simulink model "tf_hex_pos"  (R2020a)
settings: Solver=FixedStepAuto  StartTime=0.0  StopTime=10.0  FixedStep=step_size  RelTol=1e-3
values from neighbouring files (symbols this model uses):
  A = diag([Ax Ax Ax])    [tf_model_sim.m]
  g = 9.81    [tf_model_sim.m]
  m = 1.89    [tf_model_sim.m]
  pitch_tf = tf([omega_n^2], [1 2*zeta*omega_n omega_n^2])*tf([pl],[1 pl],'InputDelay',0.09)    [tf_model_sim.m]
  Ts = 0.01    [tf_model_sim.m]
undefined symbols (not defined in the file or in its folder): kd, ki, kp
settings Model: Creator=pala  LastModifiedBy=pala
settings DataIOCC: SaveFormat=StructureWithTime  ReturnWorkspaceOutputs=off

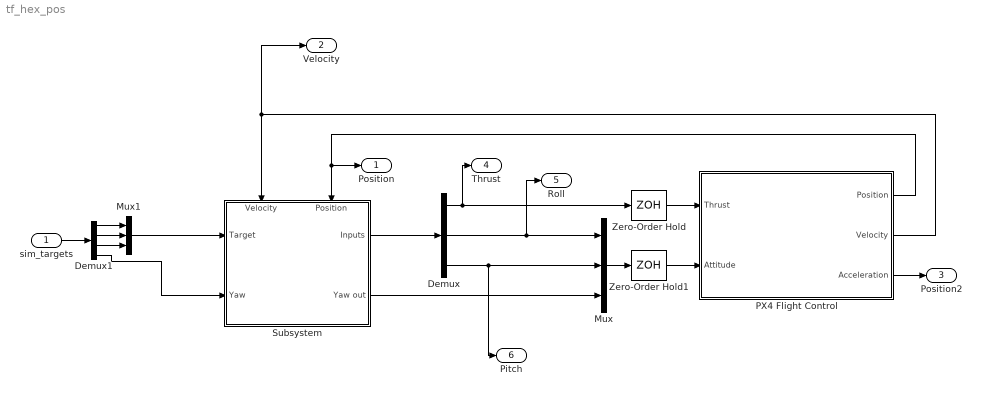
== system tf_hex_pos ==
  sim_targets : Inport
  Demux : Demux  Outputs=3
  Demux1 : Demux
  Mux : Mux  Inputs=3
  Mux1 : Mux  Inputs=3
  PX4 Flight Control : Subsystem
  Subsystem : Subsystem
      settings: PortSchema="{\"entries\":[{\"content\":{\"sides\":[{\"content\":{\"connectorIds\":[\"In1\",\"In2\"]},\"type\":\"ConnectorPlacement.EquallySpacedRectSide\",\"uuid\":\"741a1eff-fa24-40e3-8584-656dcfb9063f\"},{\"content\":{\"connectorIds\":[\"Out1\",\"Out2\"],\"side\":\"RIGHT\"},\"type\":\"ConnectorPlacement.EquallySpacedRectSide\",\"uuid\":\"ed08c2cd-e579-42d0-ad38-ef4d944c32e6\"},{\"content\":{\"connectorIds\":[\"In3\",\"In4\"],\"side\":\"TOP\"},\"type\":\"ConnectorPlacement.EquallySpacedRectSide\",\"uuid\":\"8a6d1a88-6848-4266-a6d4-735010b8417e\"}]},\"type\":\"ConnectorPlacement.EquallySpacedConnector\",\"uuid\":\"0638f19b-f024-4dd2-b120-329a1c216fc8\"}],\"packageUris\":[\"http://schema.mathworks.com/mf0/Connector/19700101\"],\"version\":\"1.0\"}"
  Zero-Order Hold : ZeroOrderHold  SampleTime=Ts
  Zero-Order Hold1 : ZeroOrderHold  SampleTime=Ts
  Position : Outport
  Velocity : Outport  Port=2
  Position2 : Outport  Port=3
  Thrust : Outport  Port=4
  Roll : Outport  Port=5
  Pitch : Outport  Port=6
  wires:
  Demux/3 -> Pitch/1, Mux/2
  Demux/2 -> Roll/1, Mux/1
  Demux/1 -> Zero-Order Hold/1, Thrust/1
  Mux/1 -> Zero-Order Hold1/1
  PX4 Flight Control/1(Position) -> Position/1, Subsystem/4(Position)
  Mux1/1 -> Subsystem/1(Target)
  PX4 Flight Control/2(Velocity) -> Velocity/1, Subsystem/3(Velocity)
  Demux1/4 -> Subsystem/2(Yaw)
  Subsystem/1(Inputs) -> Demux/1
  Subsystem/2(Yaw out) -> Mux/3
  sim_targets/1 -> Demux1/1
  Demux1/1 -> Mux1/1
  Demux1/2 -> Mux1/2
  Demux1/3 -> Mux1/3
  PX4 Flight Control/3(Acceleration) -> Position2/1
  Zero-Order Hold1/1 -> PX4 Flight Control/2(Attitude)
  Zero-Order Hold/1 -> PX4 Flight Control/1(Thrust)

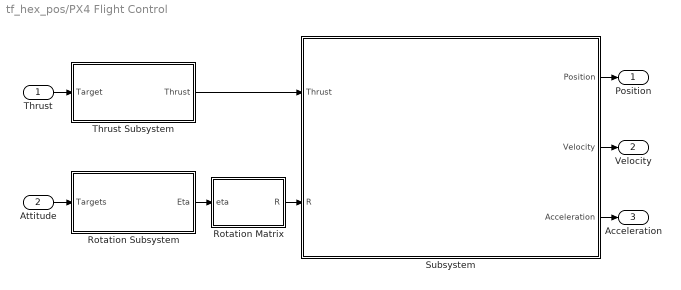
== system tf_hex_pos/PX4 Flight Control ==
  Thrust : Inport
  Attitude : Inport  Port=2
  Rotation Matrix : MATLAB Function  TreatAsAtomicUnit=on
  Rotation Subsystem : Subsystem
  Subsystem : Subsystem
  Thrust Subsystem : Subsystem
  Position : Outport
  Velocity : Outport  Port=2
  Acceleration : Outport  Port=3
  wires:
  Rotation Subsystem/1(Eta) -> Rotation Matrix/1(eta)
  Rotation Matrix/1(R) -> Subsystem/2(R)
  Subsystem/3(Acceleration) -> Acceleration/1
  Thrust/1 -> Thrust Subsystem/1(Target)
  Thrust Subsystem/1(Thrust) -> Subsystem/1(Thrust)
  Subsystem/1(Position) -> Position/1
  Subsystem/2(Velocity) -> Velocity/1
  Attitude/1 -> Rotation Subsystem/1(Targets)

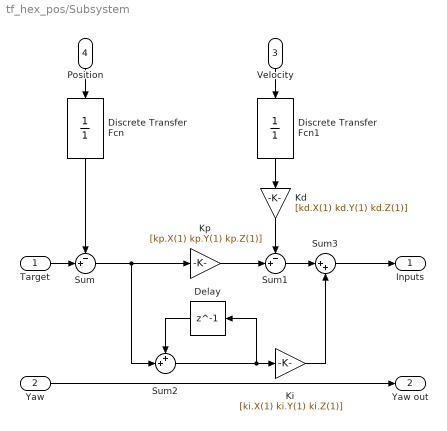
== system tf_hex_pos/Subsystem ==
  Target : Inport
  Yaw : Inport  Port=2
  Velocity : Inport  Port=3
  Position : Inport  Port=4
  Delay : Delay  DelayLength=1  SampleTime=Ts
  Discrete Transfer Fcn : DiscreteTransferFcn  Denominator=[1]  SampleTime=Ts
  Discrete Transfer Fcn1 : DiscreteTransferFcn  Denominator=[1]  SampleTime=Ts
  Kd : Gain  Gain=[kd.X(1) kd.Y(1) kd.Z(1)]
  Ki : Gain  Gain=[ki.X(1) ki.Y(1) ki.Z(1)]
  Kp : Gain  Gain=[kp.X(1) kp.Y(1) kp.Z(1)]
  Sum : Sum  Inputs=-+|
  Sum1 : Sum  Inputs=-+|
  Sum2 : Sum  Inputs=++|
  Sum3 : Sum  Inputs=|++
  Inputs : Outport
  Yaw out : Outport  Port=2
  wires:
  Target/1 -> Sum/2
  Kd/1 -> Sum1/1
  Ki/1 -> Sum3/2
  Sum/1 -> Kp/1, Sum2/2
  Position/1 -> Discrete Transfer Fcn/1
  Velocity/1 -> Discrete Transfer Fcn1/1
  Yaw/1 -> Yaw out/1
  Kp/1 -> Sum1/2
  Sum2/1 -> Ki/1, Delay/1
  Discrete Transfer Fcn1/1 -> Kd/1
  Sum3/1 -> Inputs/1
  Sum1/1 -> Sum3/1
  Discrete Transfer Fcn/1 -> Sum/1
  Delay/1 -> Sum2/1

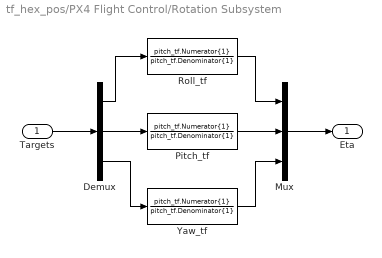
== system tf_hex_pos/PX4 Flight Control/Rotation Subsystem ==
  Targets : Inport
  Demux : Demux  Outputs=3
  Mux : Mux  Inputs=3
  Pitch_tf : TransferFcn  Numerator=pitch_tf.Numerator{1}  Denominator=pitch_tf.Denominator{1}
  Roll_tf : TransferFcn  Numerator=pitch_tf.Numerator{1}  Denominator=pitch_tf.Denominator{1}
  Yaw_tf : TransferFcn  Numerator=pitch_tf.Numerator{1}  Denominator=pitch_tf.Denominator{1}
  Eta : Outport
  wires:
  Demux/1 -> Roll_tf/1
  Demux/2 -> Pitch_tf/1
  Demux/3 -> Yaw_tf/1
  Targets/1 -> Demux/1
  Pitch_tf/1 -> Mux/2
  Roll_tf/1 -> Mux/1
  Yaw_tf/1 -> Mux/3
  Mux/1 -> Eta/1

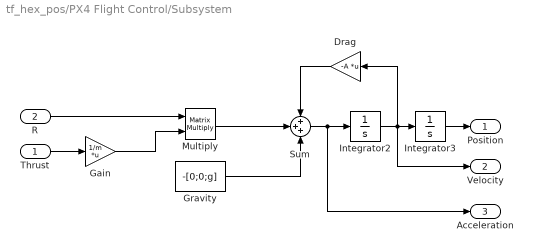
== system tf_hex_pos/PX4 Flight Control/Subsystem ==
  Thrust : Inport
  R : Inport  Port=2
  Drag : Gain  Gain=-A  Multiplication=Matrix(K*u)
  Gain : Gain  Gain=1/m  Multiplication=Matrix(K*u)
  Gravity : Constant  Value=-[0;0;g]
  Integrator2 : Integrator
  Integrator3 : Integrator
  Multiply : Product  Inputs=**  Multiplication=Matrix(*)
  Sum : Sum  Inputs=+++
  Position : Outport  VectorParamsAs1DForOutWhenUnconnected=off
  Velocity : Outport  Port=2  VectorParamsAs1DForOutWhenUnconnected=off
  Acceleration : Outport  Port=3  VectorParamsAs1DForOutWhenUnconnected=off
  wires:
  Sum/1 -> Acceleration/1, Integrator2/1
  R/1 -> Multiply/1
  Gravity/1 -> Sum/3
  Thrust/1 -> Gain/1
  Integrator3/1 -> Position/1
  Integrator2/1 -> Drag/1, Velocity/1, Integrator3/1
  Multiply/1 -> Sum/2
  Gain/1 -> Multiply/2
  Drag/1 -> Sum/1

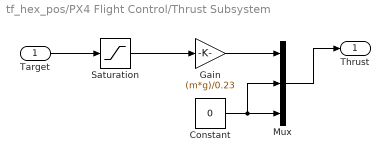
== system tf_hex_pos/PX4 Flight Control/Thrust Subsystem ==
  Target : Inport
  Constant : Constant  Value=0
  Gain : Gain  Gain=(m*g)/0.23
  Mux : Mux  Inputs=3
  Saturation : Saturate  UpperLimit=1  LowerLimit=0
  Thrust : Outport
  wires:
  Saturation/1 -> Gain/1
  Target/1 -> Saturation/1
  Gain/1 -> Mux/1
  Constant/1 -> Mux/2, Mux/3
  Mux/1 -> Thrust/1

== matlab function tf_hex_pos/PX4 Flight Control/Rotation Matrix ==
  data: eta input; R output
function R = fcn(eta)
eta_deg = rad2deg(eta);
phi     = eta_deg(1);
theta   = eta_deg(2);
psi     = eta_deg(3);

Rz = rotz(psi);
Ry = roty(theta);
Rx = rotx(phi);

R = Rz*Ry*Rx;
